simulink model "Evitaparedes"  (R2023b)
settings: Solver=VariableStepAuto  StartTime=0.0  StopTime=10.0  RelTol=1e-3
libraries: arduinolib x2
settings Model: Creator=TESTER  LastModifiedBy=TESTER

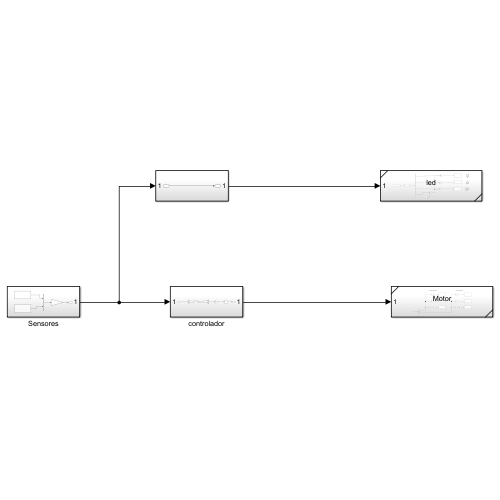
[thumbnail: Simulink's stored preview of the top-level diagram]
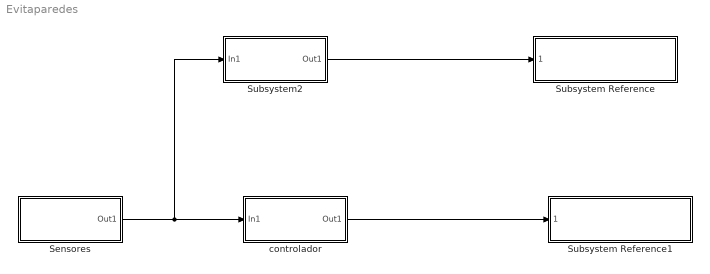
== system Evitaparedes ==
  Sensores : Subsystem
  Subsystem Reference : Subsystem  ReferencedSubsystem=led
  Subsystem Reference1 : Subsystem  ReferencedSubsystem=Motor
  Subsystem2 : Subsystem
  controlador : Subsystem
  wires:
  Sensores/1(Out1) -> Subsystem2/1(In1), controlador/1(In1)
  controlador/1(Out1) -> Subsystem Reference1/1
  Subsystem2/1(Out1) -> Subsystem Reference/1

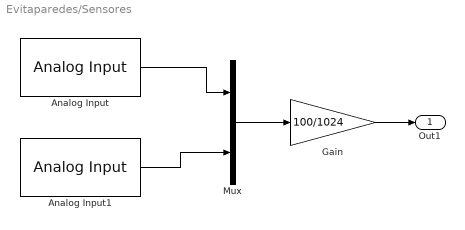
== system Evitaparedes/Sensores ==
  Analog Input : arduinolib/Analog Input  pinNumber=6  ReadResultsOnly=off  ConversionTriggerSource=Software  ExternalTriggerType=uint32( 0 )  OutputDataType=uint16  EnableConversionCompleteNotify=off  EnableOuputStatus=off  SampleTime=-1  blockPlatform=arduino
  Analog Input1 : arduinolib/Analog Input  pinNumber=8  ReadResultsOnly=off  ConversionTriggerSource=Software  ExternalTriggerType=uint32( 0 )  OutputDataType=uint16  EnableConversionCompleteNotify=off  EnableOuputStatus=off  SampleTime=-1  blockPlatform=arduino
  Gain : Gain  Gain=100/1024
  Mux : Mux  Inputs=2
  Out1 : Outport
  wires:
  Analog Input/1 -> Mux/1
  Mux/1 -> Gain/1
  Gain/1 -> Out1/1
  Analog Input1/1 -> Mux/2

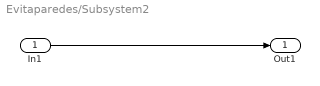
== system Evitaparedes/Subsystem2 ==
  In1 : Inport
  Out1 : Outport
  wires:
  In1/1 -> Out1/1

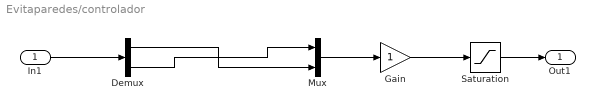
== system Evitaparedes/controlador ==
  In1 : Inport
  Demux : Demux  Outputs=2
  Gain : Gain
  Mux : Mux  Inputs=2
  Saturation : Saturate
  Out1 : Outport
  wires:
  Demux/1 -> Mux/2
  Demux/2 -> Mux/1
  Gain/1 -> Saturation/1
  Mux/1 -> Gain/1
  In1/1 -> Demux/1
  Saturation/1 -> Out1/1
